simulink model "filter"  (R2017b)
settings: Solver=ode45  StartTime=0.0  StopTime=10.0  RelTol=1e-3  EnableMultiTasking=on
libraries: dspvision x1, dspobslib x1
settings Model: Creator=erfan  LastModifiedBy=microsoft
settings DataIOCC: LimitDataPoints=on  SaveFormat=Array
settings OptimizationCC: LifeSpan=inf
settings DebuggingCC: SFUnexpectedBacktrackingDiag=warning  SFNoUnconditionalDefaultTransitionDiag=warning  SFExecutionAtInitializationDiag=none
settings HardwareCC: ProdBitPerPointer=32  ProdBitPerSizeT=32  ProdBitPerPtrDiffT=32  ProdLargestAtomicFloat=None  ProdIntDivRoundTo=Undefined  ProdEndianess=Unspecified  ProdWordSize=32  ProdHWDeviceType=32-bit Generic
settings ModelReferenceCC: PropagateSignalLabelsOutOfModel=off
settings CodeAppCC: StateflowObjectComments=on
settings GRTTargetCC: TargetLangStandard=C89/C90 (ANSI)  GeneratePreprocessorConditionals=Disable all
settings ConfigComp: CovMetricSettings=dw  CovHtmlReporting=on  CovSaveCumulativeToWorkspaceVar=on  CovSaveSingleToWorkspaceVar=on  CovExternalEMLEnable=off

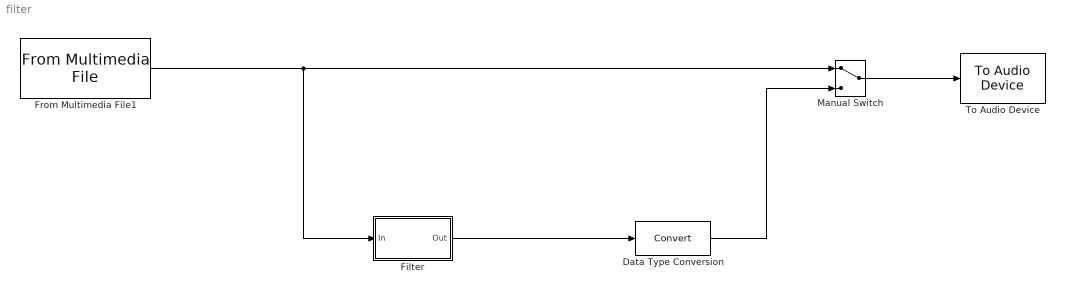
== system filter ==
  Data Type Conversion : DataTypeConversion
  Filter : Subsystem  Tag=BlockMethodSubSystem
  From Multimedia File1 : dspvision/From Multimedia File  inputFilename=C:\Users\microsoft\Documents\UT\FPGA\Lab3\lab3\matlab_files\input.wav  loop=on  numPlays=inf  outputStreams=Audio only  videoDataType=single  audioDataType=double  inheritSampleTime=on  userDefinedSampleTime=1/30  noAudioOutput=off  isIntensityVideo=off  fourcc=RGB  colorVideoFormat=Separate color signals  outputEOF=off  dataOrg=Column-major  audioFrameSize=1024  computeAudioFrameSize=off  outSamplingMode=Sample based
      settings: SourceProductBaseCode=VP
  Manual Switch : ManualSwitch
  To Audio Device : dspobslib/To Audio Device  deviceName=Default  inheritSampleRate=on  sampleRate=44100  deviceDatatype=Determine from input data type  autoBufferSize=on  bufferSize=4096  queueDuration=1.0  defaultOutputChannelMapping=on  outputChannelMapping=1:2  outputNumUnderrunSamples=off
      settings: SourceProductName=DSP System Toolbox  SourceProductBaseCode=DS
  wires:
  Filter/1(Out) -> Data Type Conversion/1
  From Multimedia File1/1 -> Filter/1(In), Manual Switch/1
  Data Type Conversion/1 -> Manual Switch/2
  Manual Switch/1 -> To Audio Device/1

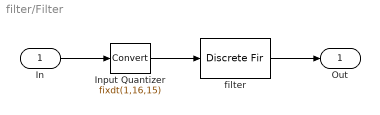
== system filter/Filter ==
  In : Inport
  Input Quantizer : DataTypeConversion  OutDataTypeStr=fixdt(1,16,15)  RndMeth=Round  SaturateOnIntegerOverflow=on
  filter : DiscreteFir  Coefficients=[0.0036840626645888849 0.0029312178951941743 -0.0016555557872138787 -0.0094658006262221487 -0.014728988749761765 -0.012043455818540919 -0.0024153450486515335 0.0061508974886797865 0.0057346838199391972 -0.0029869837480845968 -0.010248646060759582 -0.0069100677011288292 0.0049600833394223623 0.012760498811448804 0.0064944265875801366 -0.0088578127181410844 -0.016509451051346109 -0.0056917444325811067 0.014275137848099114 0.021094777907581318 0.0035477963062536225 -0.022583814488611353 -0.027290637336714385 0.0009899428770668451 0.036622083754008841 0.037080022397728479 -0.011323602667843838 -0.067118307765611007 -0.059898345240720782 0.046659400825621734 0.2109817865590492 0.33423543383381704 0.33423543383381704 0.2109817865590492 0.046659400825621734 -0.059898345240720782 -0.067118307765611007 -0.011323602667843838 0.037080022397728479 0.036622083754008841 0.0009899428770668451 -0.027290637336714385 -0.022583814488611353 0.0035477963062536225 0.021094777907581318 0.014275137848099114 -0.0056917444325811067 -0.016509451051346109 -0.0088578127181410844 0.0064944265875801366 0.012760498811448804 0.0049600833394223623 -0.0069100677011288292 -0.010248646060759582 -0.0029869837480845968 0.0057346838199391972 0.0061508974886797865 -0.0024153450486515335 -0.012043455818540919 -0.014728988749761765 -0.0094658006262221487 -0.0016555557872138787 0.0029312178951941743 0.0036840626645888849]  InputProcessing=Columns as channels (frame based)  CoefDataTypeStr=fixdt(true,16,16)  ProductDataTypeStr=fixdt(true,31,31)  AccumDataTypeStr=fixdt(true,34,31)  OutDataTypeStr=fixdt(true,34,31)  RndMeth=Convergent
  Out : Outport
  wires:
  In/1 -> Input Quantizer/1
  Input Quantizer/1 -> filter/1
  filter/1 -> Out/1
